simulink model "adc_demo"  (Simulink 8.3)
settings: Solver=VariableStepDiscrete  StartTime=0.0  StopTime=1  RelTol=1e-3
libraries: simulink_extras x1
settings Model: Creator=rcheng  LastModifiedBy=rodralez  CovHtmlReporting=off
settings OptimizationCC: ExpressionDepthLimit=2147483647  InitFltsAndDblsToZero=on
settings DebuggingCC: FcnCallInpInsideContextMsg=EnableAllAsWarning  FrameProcessingCompatibilityMsg=error

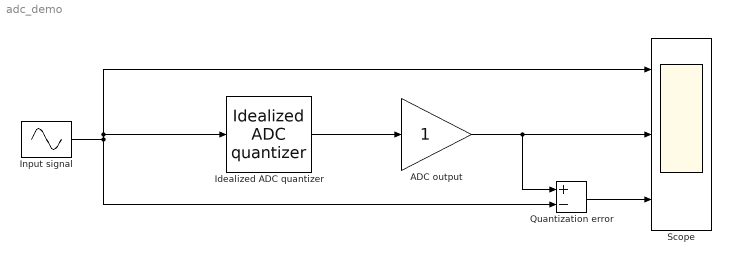
== system adc_demo ==
  ADC output : Gain
  Idealized ADC quantizer : simulink_extras/Additional Discrete/Idealized ADC quantizer  NumberOfConverterBits=16  Vmin=0  Vmax=5  OutputDataType=int16  OutputNegativeValues=on
  Input signal : Sin  Amplitude=2.5  Frequency=2*pi*100  SampleTime=1/10000
  Quantization error : Sum  Inputs=+-
  Scope : Scope  NumInputPorts=3
      settings: TimeRange=0.5  ShowLegends=on  LimitDataPoints=on  MaxDataPoints=5000  SaveName=ScopeData  YMin=-3.125~-36864.00000~-36863.6875  YMax=3.125~4096.00000~4093.1875  SampleTime=-1
  wires:
  Quantization error/1 -> Scope/3
  Idealized ADC quantizer/1 -> ADC output/1
  ADC output/1 -> Quantization error/1, Scope/2
  Input signal/1 -> Idealized ADC quantizer/1, Scope/1, Quantization error/2
